simulink model "Projekt_Kessel_ungesteuert"  (Simulink 4.00)
settings: Solver=ode45  StartTime=0.0  StopTime=inf  RelTol=1e-3
libraries: simulink3 x8
settings Model: LastModifiedBy=Administrator  BlockReductionOpt=off

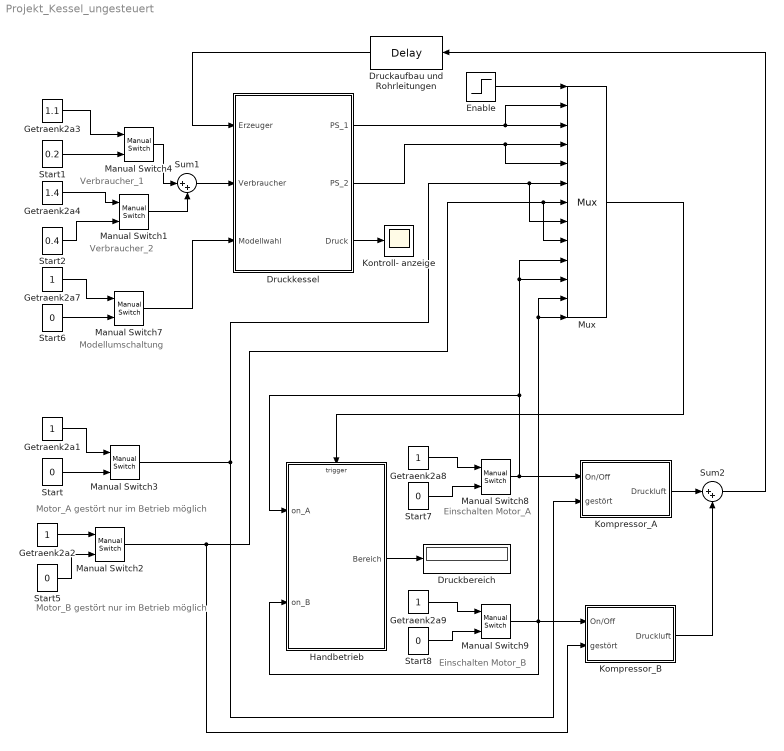
== system Projekt_Kessel_ungesteuert ==
  note: Motor_A gestört nur im Betrieb möglich
  note: Verbraucher_1
  note: Verbraucher_2
  note: Motor_B gestört nur im Betrieb möglich
  note: Modellumschaltung
  note: Einschalten Motor_A
  note: Einschalten Motor_B
  Druckaufbau und Rohrleitungen : TransportDelay  Orientation=left  DelayTime=2  InitialInput=0  BufferSize=1024  PadeOrder=0
  Druckbereich : Display
      settings: Format=short
  Druckkessel : Subsystem
      settings: RTWFcnNameOpts=Auto  RTWFileNameOpts=Auto
  Enable : Step  Time=0.5  Before=0  After=1  SampleTime=0
  Getraenk2a{1..2,7..9} (5 alike) : Constant  Value=1
  Getraenk2a3 : Constant  Value=1.1
  Getraenk2a4 : Constant  Value=1.4
  Handbetrieb : Stateflow chart  TreatAsAtomicUnit=on
      settings: RTWFcnNameOpts=Auto  RTWFileNameOpts=Auto
  Kompressor_A : Subsystem
      settings: RTWFcnNameOpts=Auto  RTWFileNameOpts=Auto
  Kompressor_B : Subsystem
      settings: RTWFcnNameOpts=Auto  RTWFileNameOpts=Auto
  Kontroll- anzeige : Scope
      settings: TimeRange=10  YMin=4.5425  YMax=4.575  SaveToWorkspace=off  SaveName=ScopeData  LimitDataPoints=on  MaxDataPoints=5000
  Manual Switch1 : simulink3/Nonlinear/Manual Switch  sw=1  action=0
  Manual Switch{2..4,8..9} (5 alike) : simulink3/Nonlinear/Manual Switch  sw=0  action=0
  Manual Switch7 : simulink3/Nonlinear/Manual Switch  sw=1  action=0
  Mux : Mux  Inputs=13
      settings: DisplayOption=none
  Start{,5..8} (5 alike) : Constant  Value=0
  Start1 : Constant  Value=0.2
  Start2 : Constant  Value=0.4
  Sum1 : Sum  Inputs=|++  SaturateOnIntegerOverflow=on
  Sum2 : Sum  Inputs=|++  SaturateOnIntegerOverflow=on
  wires:
  Enable/1 -> Mux/1
  Mux/1 -> Handbetrieb/Trigger
  Start5/1 -> Manual Switch2/2
  Getraenk2a2/1 -> Manual Switch2/1
  Start/1 -> Manual Switch3/2
  Getraenk2a1/1 -> Manual Switch3/1
  Start1/1 -> Manual Switch4/2
  Getraenk2a3/1 -> Manual Switch4/1
  Start2/1 -> Manual Switch1/2
  Kompressor_A/1(Druckluft) -> Sum2/1
  Druckaufbau und Rohrleitungen/1 -> Druckkessel/1(Erzeuger)
  Sum2/1 -> Druckaufbau und Rohrleitungen/1
  Manual Switch3/1 -> Mux/6, Mux/8, Kompressor_A/2(gestört)
  Manual Switch2/1 -> Mux/7, Mux/9, Kompressor_B/2(gestört)
  Druckkessel/3(Druck) -> Kontroll- anzeige/1
  Start6/1 -> Manual Switch7/2
  Getraenk2a7/1 -> Manual Switch7/1
  Start7/1 -> Manual Switch8/2
  Getraenk2a8/1 -> Manual Switch8/1
  Manual Switch8/1 -> Kompressor_A/1(On/Off), Mux/10, Mux/11, Handbetrieb/1(on_A)
  Handbetrieb/1(Bereich) -> Druckbereich/1
  Kompressor_B/1(Druckluft) -> Sum2/2
  Start8/1 -> Manual Switch9/2
  Getraenk2a9/1 -> Manual Switch9/1
  Druckkessel/1(PS_1) -> Mux/2, Mux/3
  Druckkessel/2(PS_2) -> Mux/4, Mux/5
  Manual Switch9/1 -> Mux/12, Mux/13, Kompressor_B/1(On/Off), Handbetrieb/2(on_B)
  Getraenk2a4/1 -> Manual Switch1/1
  Manual Switch7/1 -> Druckkessel/3(Modellwahl)
  Sum1/1 -> Druckkessel/2(Verbraucher)
  Manual Switch1/1 -> Sum1/2
  Manual Switch4/1 -> Sum1/1

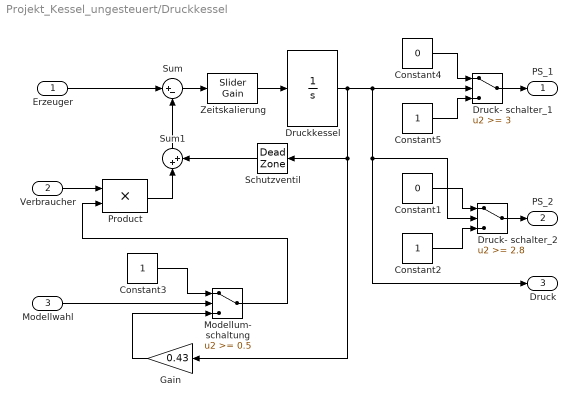
== system Projekt_Kessel_ungesteuert/Druckkessel ==
  Erzeuger : Inport  Port=1
  Verbraucher : Inport  Port=2
  Modellwahl : Inport  Port=3
  Constant1 : Constant  Value=0
  Constant2 : Constant  Value=1
  Constant3 : Constant  Value=1
  Constant4 : Constant  Value=0
  Constant5 : Constant  Value=1
  Druck- schalter_1 : Switch  Threshold=3
  Druck- schalter_2 : Switch  Threshold=2.8
  Druckkessel : Integrator  ExternalReset=none  InitialConditionSource=internal  InitialCondition=3.5  LimitOutput=on  UpperSaturationLimit=10  LowerSaturationLimit=0  ShowSaturationPort=off  ShowStatePort=off  AbsoluteTolerance=auto
  Gain : Gain  Orientation=left  Gain=0.43  Multiplication=Element-wise(K.*u)  SaturateOnIntegerOverflow=on
  Modellum- schaltung : Switch  Threshold=0.5
  Product : Product  Inputs=2  Multiplication=Element-wise(.*)  SaturateOnIntegerOverflow=on
  Schutzventil : DeadZone  Orientation=left  LowerValue=-1.  UpperValue=5  SaturateOnIntegerOverflow=on  LinearizeAsGain=on
  Sum : Sum  Inputs=|+-  SaturateOnIntegerOverflow=on
  Sum1 : Sum  Orientation=up  Inputs=|++  SaturateOnIntegerOverflow=on
  Zeitskalierung : simulink3/Math/Slider Gain  low=0  gain=0.001  high=0.2
  PS_1 : Outport  Port=1
  PS_2 : Outport  Port=2
  Druck : Outport  Port=3
  wires:
  Druckkessel/1 -> Druck- schalter_1/2, Druck- schalter_2/2, Druck/1, Schutzventil/1, Gain/1
  Constant4/1 -> Druck- schalter_1/1
  Constant5/1 -> Druck- schalter_1/3
  Druck- schalter_1/1 -> PS_1/1
  Constant1/1 -> Druck- schalter_2/1
  Constant2/1 -> Druck- schalter_2/3
  Druck- schalter_2/1 -> PS_2/1
  Sum/1 -> Zeitskalierung/1
  Zeitskalierung/1 -> Druckkessel/1
  Verbraucher/1 -> Product/1
  Schutzventil/1 -> Sum1/2
  Sum1/1 -> Sum/2
  Product/1 -> Sum1/1
  Modellwahl/1 -> Modellum- schaltung/2
  Constant3/1 -> Modellum- schaltung/1
  Modellum- schaltung/1 -> Product/2
  Erzeuger/1 -> Sum/1
  Gain/1 -> Modellum- schaltung/3

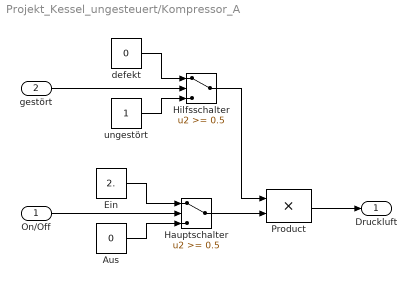
== system Projekt_Kessel_ungesteuert/Kompressor_A ==
  On/Off : Inport  Port=1
  gestört : Inport  Port=2
  Aus : Constant  Value=0
  Ein : Constant  Value=2.
  Hauptschalter : Switch  Threshold=0.5
  Hilfsschalter : Switch  Threshold=0.5
  Product : Product  Inputs=2  Multiplication=Element-wise(.*)  SaturateOnIntegerOverflow=on
  defekt : Constant  Value=0
  ungestört : Constant  Value=1
  Druckluft : Outport  Port=1
  wires:
  Ein/1 -> Hauptschalter/1
  Aus/1 -> Hauptschalter/3
  On/Off/1 -> Hauptschalter/2
  defekt/1 -> Hilfsschalter/1
  ungestört/1 -> Hilfsschalter/3
  gestört/1 -> Hilfsschalter/2
  Hauptschalter/1 -> Product/2
  Product/1 -> Druckluft/1
  Hilfsschalter/1 -> Product/1

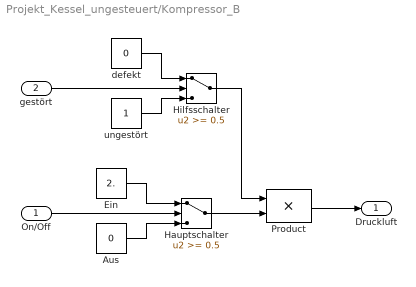
== system Projekt_Kessel_ungesteuert/Kompressor_B ==
  On/Off : Inport  Port=1
  gestört : Inport  Port=2
  Aus : Constant  Value=0
  Ein : Constant  Value=2.
  Hauptschalter : Switch  Threshold=0.5
  Hilfsschalter : Switch  Threshold=0.5
  Product : Product  Inputs=2  Multiplication=Element-wise(.*)  SaturateOnIntegerOverflow=on
  defekt : Constant  Value=0
  ungestört : Constant  Value=1
  Druckluft : Outport  Port=1
  wires:
  Ein/1 -> Hauptschalter/1
  Aus/1 -> Hauptschalter/3
  On/Off/1 -> Hauptschalter/2
  defekt/1 -> Hilfsschalter/1
  ungestört/1 -> Hilfsschalter/3
  gestört/1 -> Hilfsschalter/2
  Hauptschalter/1 -> Product/2
  Product/1 -> Druckluft/1
  Hilfsschalter/1 -> Product/1

== stateflow chart Handbetrieb ==
  state Kessel [parallel]
    state Druck_hoch
      entry:Bereich=3;
    state Druck_mittel
      en:Bereich=2;
    state Druck_tief
      en:Bereich=1;
    Druck_hoch -> Druck_mittel : PS_1_s
    Druck_mittel -> Druck_tief : PS_2_s
    Druck_tief -> Druck_mittel : PS_2_f
    Druck_mittel -> Druck_hoch : PS_1_f
    (default) -> Druck_hoch
  state Motor_A [parallel]
    state Off
    state On
    state Down
    Motor_A.Off -> Motor_A.On : Ein_A
    Motor_A.Down -> (junction 15) : OK_A
    (default) -> Motor_A.Off
    Motor_A.On -> Motor_A.Off : Aus_A
    Motor_A.On -> Motor_A.Down : Down_A
    (junction 15) -> Motor_A.Off
    (junction 15) -> Motor_A.On : [on_A==1]
  state Motor_B [parallel]
    state On
    state Off
    state Down
    Motor_B.On -> Motor_B.Off : Aus_B
    Motor_B.On -> Motor_B.Down : Down_B
    Motor_B.Off -> Motor_B.On : Ein_B
    (junction 16) -> Motor_B.On : [on_B==1]
    (default) -> Motor_B.Off
    (junction 16) -> Motor_B.Off
    Motor_B.Down -> (junction 16) : OK_B
  (default) -> Kessel
  (default) -> Motor_A
  (default) -> Motor_B
  data: Bereich output int16 =3; on_A input int16; on_B input int16
  events: Enable input RISING_EDGE_EVENT; PS_1_s input RISING_EDGE_EVENT; PS_1_f input FALLING_EDGE_EVENT; PS_2_s input RISING_EDGE_EVENT; PS_2_f input FALLING_EDGE_EVENT; Down_A input RISING_EDGE_EVENT; Down_B input RISING_EDGE_EVENT; OK_A input FALLING_EDGE_EVENT; OK_B input FALLING_EDGE_EVENT; Ein_A input RISING_EDGE_EVENT; Aus_A input FALLING_EDGE_EVENT; Ein_B input RISING_EDGE_EVENT; Aus_B input FALLING_EDGE_EVENT
